simulink model "mlf_cast_"  (R2015b)
settings: Solver=FixedStepDiscrete  SolverMode=SingleTasking  StartTime=0.0  StopTime=4  RelTol=1e-3
libraries: simulink x1
settings Model: Creator=at-mt  LastModifiedBy=amatsumo
settings DataIOCC: SaveFormat=Array  SignalLoggingSaveFormat=ModelDataLogs  SaveOutput=off  SignalLogging=off  SaveTime=off
settings OptimizationCC: BlockReduction=off  ConditionallyExecuteInputs=off  DefaultParameterBehavior=Inlined  ExpressionDepthLimit=2147483647
settings DebuggingCC: AlgebraicLoopMsg=error  UnderspecifiedInitializationDetection=Classic  MergeDetectMultiDrivingBlocksExec=none  SolverPrmCheckMsg=warning  SingleTaskRateTransMsg=error  FcnCallInpInsideContextMsg=UseLocalSettings  StateNameClashWarn=warning
settings HardwareCC: ProdBitPerPointer=32  ProdLargestAtomicFloat=None  ProdIntDivRoundTo=Undefined  ProdEndianess=Unspecified  ProdWordSize=32  ProdHWDeviceType=ASIC/FPGA->ASIC/FPGA  ProdEqTarget=off
settings GRTTargetCC: GeneratePreprocessorConditionals=Disable all  CombineOutputUpdateFcns=off  GRTInterface=on
settings ConfigComp: CovModelRefEnable=Off  CovSFcnEnable=off

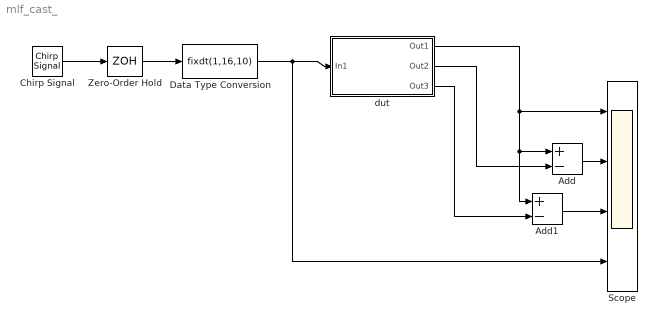
== system mlf_cast_ ==
  Add : Sum  Inputs=+-
  Add1 : Sum  Inputs=+-
  Chirp Signal : simulink/Sources/Chirp Signal  f1=10  T=10  f2=500
  Data Type Conversion : DataTypeConversion  OutDataTypeStr=fixdt(1,16,10)
  Scope : Scope  NumInputPorts=4
  Zero-Order Hold : ZeroOrderHold  SampleTime=1/1000
  dut : Subsystem
  wires:
  Chirp Signal/1 -> Zero-Order Hold/1
  Zero-Order Hold/1 -> Data Type Conversion/1
  Data Type Conversion/1 -> Scope/4, dut/1(In1)
  dut/1(Out1) -> Add1/1, Add/1, Scope/1
  Add/1 -> Scope/2
  dut/2(Out2) -> Add/2
  Add1/1 -> Scope/3
  dut/3(Out3) -> Add1/2

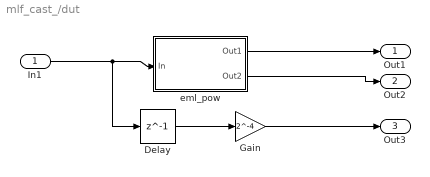
== system mlf_cast_/dut ==
  In1 : Inport
  Delay : Delay  DelayLength=1
  Gain : Gain  Gain=2^-4
  eml_pow : MATLAB Function  TreatAsAtomicUnit=on
  Out1 : Outport
  Out2 : Outport  Port=2
  Out3 : Outport  Port=3
  wires:
  In1/1 -> Delay/1, eml_pow/1(In)
  eml_pow/1(Out1) -> Out1/1
  eml_pow/2(Out2) -> Out2/1
  Gain/1 -> Out3/1
  Delay/1 -> Gain/1

== matlab function mlf_cast_/dut/eml_pow ==
  settings: fimath=|
      | fimath(...
      | 'RoundMode', 'floor',...
      | 'OverflowMode', 'wrap',...
      | 'ProductMode', 'KeepLSB', 'ProductWordLength', 16,...
      | 'SumMode', 'KeepLSB', 'SumWordLength', 16,...
      | 'CastBeforeSum', true)
  data: In input; Out1 output; Out2 output
function [Out1,Out2] = fcn(In)

% nt_in = numerictype(In);
nt_in = numerictype(1, 16, 14);
persistent buf1 buf2
if isempty(buf1)||isempty(buf2)
	buf1 = fi(0, nt_in);
	buf2 = fi(0, nt_in);
	
end

Out1 = buf1;
Out2 = buf2;

% buf1 = fi(In*fi(2^-4, 0, 4, 4), nt_in);
buf1 = cast(In*fi(2^-4, 0, 4, 4), 'like', buf1);
buf2 = fi(In*fi(0.0625, 0, 4, 4), nt_in);
% buf1 = fi(In*(2^-4), 1, 16, 14);
% buf2 = fi(In*0.0625, 1, 16, 14);
